simulink model "Simulation_of_Pendulum"  (R2022b)
settings: Solver=ode4  StartTime=0.0  StopTime=30  FixedStep=0.001  RelTol=1e-3
values from neighbouring files (symbols this model uses):
  K = lqr(A,B,Q,R)    [lqr_cartpend.m]
settings Model: Creator=sokse  LastModifiedBy=sokse

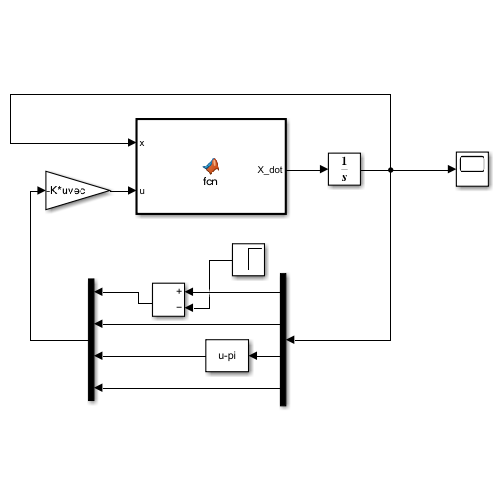
[thumbnail: Simulink's stored preview of the top-level diagram]
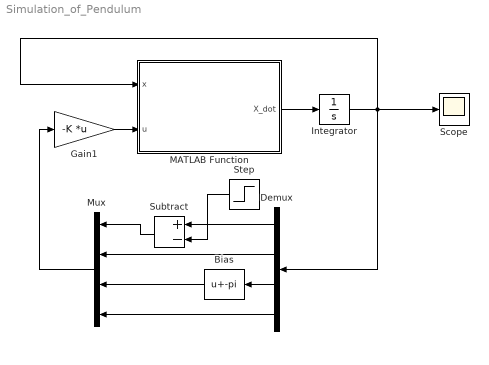
== system Simulation_of_Pendulum ==
  Bias : Bias  Bias=-pi  SaturateOnIntegerOverflow=off
  Demux : Demux
  Gain1 : Gain  Gain=-K  Multiplication=Matrix(K*u) (u vector)
  Integrator : Integrator  InitialCondition=[0;0;pi;0]
  MATLAB Function : MATLAB Function  TreatAsAtomicUnit=on
  Mux : Mux
  Scope : Scope
  Step : Step  Time=10  SampleTime=0
  Subtract : Sum  Inputs=+-
  wires:
  MATLAB Function/1(X_dot) -> Integrator/1
  Integrator/1 -> Demux/1, MATLAB Function/1(x), Scope/1
  Gain1/1 -> MATLAB Function/2(u)
  Demux/3 -> Bias/1
  Demux/1 -> Subtract/1
  Step/1 -> Subtract/2
  Subtract/1 -> Mux/1
  Demux/2 -> Mux/2
  Bias/1 -> Mux/3
  Demux/4 -> Mux/4
  Mux/1 -> Gain1/1

== matlab function Simulation_of_Pendulum/MATLAB Function ==
  data: x input; u input; X_dot output
function X_dot = fcn(x,u)

m = 1;
M = 5;
L = 2;
g = -10;
d = 1;


s = 1; % pendulum up (s=1)

A = [0 1 0 0;
    0 -d/M -m*g/M 0;
    0 0 0 1;
    0 -s*d/(M*L) -s*(m+M)*g/(M*L) 0];

B = [0; 1/M; 0; s*1/(M*L)];

X_dot = A*x + B*u;
